simulink model "PD_controller"  (R2019a)
settings: Solver=VariableStepAuto  StartTime=0.0  StopTime=100  RelTol=1e-3
values from neighbouring files (symbols this model uses):
  g = 9.81    [Data.m]    (also in func.m; myTransitionFcn.m)
  m = 0.1    [Data.m]    (also in myTransitionFcn.m)
  r = 0.1    [Data.m]    (also in func.m; myTransitionFcn.m)
  R = 1    [Data.m]    (also in func.m; myTransitionFcn.m)
libraries: simulink x1
settings Model: Creator=Dell  LastModifiedBy=Dell

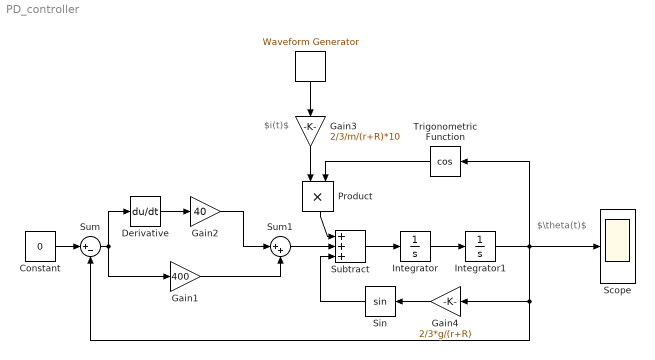
== system PD_controller ==
  note: $i(t)$
  note: $\theta(t)$
  " " : simulink/Sources/Waveform Generator  OutMin=[]  OutMax=[]  OutDataTypeStr=double  SelectedSignal=1  Signals=step()  BlockNames=MultiportSwitch_8c7b78d12e5b405  SampleTime=0.1
      settings: SourceProductName=Simulink
  Constant : Constant  Value=0
  Derivative : Derivative
  Gain1 : Gain  Gain=400
  Gain2 : Gain  Gain=40
  Gain3 : Gain  Gain=2/3/m/(r+R)*10
  Gain4 : Gain  Gain=2/3*g/(r+R)
  Integrator : Integrator
  Integrator1 : Integrator
  Product : Product
  Scope : Scope
  Sin : Trigonometry
  Subtract : Sum  Inputs=+++
  Sum : Sum  Inputs=|+-
  Sum1 : Sum  Inputs=|++
  Trigonometric Function : Trigonometry  Operator=cos
  wires:
  Sum1/1 -> Subtract/2
  Integrator1/1 -> Gain4/1, Sum/2, Scope/1, Trigonometric Function/1
  " "/1 -> Gain3/1
  Constant/1 -> Sum/1
  Sum/1 -> Derivative/1, Gain1/1
  Subtract/1 -> Integrator/1
  Gain4/1 -> Sin/1
  Trigonometric Function/1 -> Product/2
  Sin/1 -> Subtract/3
  Gain3/1 -> Product/1
  Integrator/1 -> Integrator1/1
  Product/1 -> Subtract/1
  Derivative/1 -> Gain2/1
  Gain2/1 -> Sum1/1
  Gain1/1 -> Sum1/2
